simulink model "demoCS2"  (Simulink 6.6)
settings: Solver=ode45  StartTime=0.0  StopTime=200  RelTol=1e-3
libraries: marine_gnc x5, simulink_extras x4, simulink x3
settings Model: Creator=Thor  LastModifiedBy=Thor
settings DataIOCC: SignalLoggingName=sigsOut
settings DebuggingCC: SignalResolutionControl=TryResolveAllWithWarning  SolverPrmCheckMsg=none  MultiTaskDSMMsg=warning  MultiTaskCondExecSysMsg=none  StrictBusMsg=None
settings HardwareCC: TargetUnknown=on
settings RTWCC: IncludeERTFirstTime=on
settings CodeAppCC: IgnoreCustomStorageClasses=off
settings GRTTargetCC: ModelReferenceCompliant=off  MatFileLogging=off

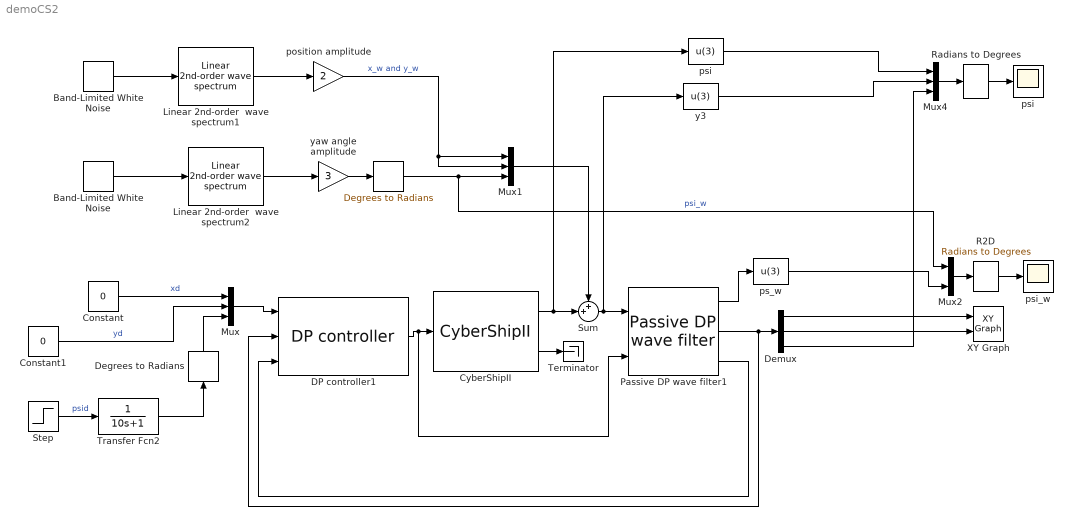
== system demoCS2 ==
  "   " : simulink_extras/Transformations/Degrees to Radians  SystemSampleTime=-1
  Band-Limited White Noise : simulink/Sources/Band-Limited White Noise  SystemSampleTime=-1  Cov=[1]  Ts=0.1  seed=[23341]
  "Band-Limited White Noise  " : simulink/Sources/Band-Limited White Noise  SystemSampleTime=-1  Cov=[1]  Ts=0.1  seed=[23341]
  Constant : Constant  Value=0
  Constant1 : Constant  Value=0
  CyberShipII : marine_gnc/Examples/Vessels/CyberShipII  SystemSampleTime=-1
  DP controller1 : marine_gnc/Control/Dynamic  Positioning /DP controller  SystemSampleTime=-1  Kp="(0.1)^2*[25.8000 0  0;  0  33.8000  1.0115;  0  1.0115  2.7600 ]"  Kd="2*0.8*0.1*[25.8000 0  0;  0  33.8000  1.0115;  0  1.0115  2.7600 ]"  Ki="(0.1^3/10)*[25.8000 0  0;  0  33.8000  1.0115;  0  1.0115  2.7600 ]"
  Degrees to Radians : simulink_extras/Transformations/Degrees to Radians  Orientation=up  SystemSampleTime=-1
  Demux : Demux  Outputs=3
  Linear 2nd-order  wave spectrum1 : marine_gnc/Environment/Waves/Linear 2nd-order  wave spectrum  SystemSampleTime=-1  sigma=0.5  w_0=0.8  lambda=0.1
  Linear 2nd-order  wave spectrum2 : marine_gnc/Environment/Waves/Linear 2nd-order  wave spectrum  SystemSampleTime=-1  sigma=0.5  w_0=0.8  lambda=0.1
  Mux : Mux  Inputs=3
  Mux1 : Mux  Inputs=3
  Mux2 : Mux  Inputs=2
  Mux4 : Mux  Inputs=3
  Passive DP wave filter1 : marine_gnc/Navigation/Observers/Passive DP wave filter  SystemSampleTime=-1  lambda=0.1*diag([1 1 1])  w_o=diag([0.8 0.8 0.8])  K4=0.1*diag([1 1 0.1])  K3=0.1*diag([1 1 0.1])  w_c=1.3*diag([0.8 0.8 0.8])  T_b=diag([100 100 100])  M="[ 25.8000   0    0;   0   33.8000   1.0115; 0   1.0115    2.7600 ]"  D="[2 0  0;  0 7 0.1; 0 0.1 0.5]"
  R2D : simulink_extras/Transformations/Radians to Degrees  SystemSampleTime=-1
  Radians to Degrees : simulink_extras/Transformations/Radians to Degrees  SystemSampleTime=-1
  Step : Step  Time=30  After=10  SampleTime=0
  "Sum  " : Sum  Inputs=++|  SaturateOnIntegerOverflow=on  InputSameDT=on
  Terminator : Terminator
  Transfer Fcn2 : TransferFcn  Denominator=[10 1]
  XY Graph : simulink/Sinks/XY Graph  SystemSampleTime=-1  xmin=-10  xmax=10  ymin=-10  ymax=10  st=-1
  "position amplitude " : Gain  Gain=2  SaturateOnIntegerOverflow=on
  ps_w : Fcn  Expr=u(3)
  psi : Fcn  Expr=u(3)
  "psi  " : Scope
      settings: TimeRange=200  YMax=20
  psi_w : Scope
      settings: TimeRange=200  YMin=-6  YMax=6
  y3 : Fcn  Expr=u(3)
  yaw angle amplitude : Gain  Gain=3  SaturateOnIntegerOverflow=on
  wires:
  Constant/1 -> Mux/1  "xd"
  Step/1 -> Transfer Fcn2/1  "psid"
  Degrees to Radians/1 -> Mux/3
  Constant1/1 -> Mux/2  "yd"
  Demux/1 -> XY Graph/1
  Demux/2 -> XY Graph/2
  Mux/1 -> DP controller1/1
  Transfer Fcn2/1 -> Degrees to Radians/1
  Band-Limited White Noise/1 -> Linear 2nd-order  wave spectrum2/1
  Linear 2nd-order  wave spectrum2/1 -> yaw angle amplitude/1
  yaw angle amplitude/1 -> "   "/1
  "Band-Limited White Noise  "/1 -> Linear 2nd-order  wave spectrum1/1
  Linear 2nd-order  wave spectrum1/1 -> "position amplitude "/1
  "position amplitude "/1 -> Mux1/2, Mux1/1  "x_w and y_w"
  "   "/1 -> Mux1/3, Mux2/1  "psi_w"
  Mux1/1 -> "Sum  "/1
  CyberShipII/1 -> "Sum  "/2, psi/1
  Mux2/1 -> R2D/1
  "Sum  "/1 -> y3/1, Passive DP wave filter1/1
  Radians to Degrees/1 -> "psi  "/1
  CyberShipII/2 -> Terminator/1
  R2D/1 -> psi_w/1
  ps_w/1 -> Mux2/2
  Mux4/1 -> Radians to Degrees/1
  Demux/3 -> Mux4/3
  y3/1 -> Mux4/2
  psi/1 -> Mux4/1
  Passive DP wave filter1/2 -> Demux/1, DP controller1/2
  Passive DP wave filter1/1 -> ps_w/1
  DP controller1/1 -> CyberShipII/1, Passive DP wave filter1/2
  Passive DP wave filter1/3 -> DP controller1/3
